simulink model "Passive_Balance"  (R2020a)
settings: Solver=FixedStepDiscrete  StartTime=0.0  StopTime=1  FixedStep=1e-3  RelTol=1e-3
libraries: simulink x1
settings Model: Creator=Administrator  LastModifiedBy=Administrator
settings OptimizationCC: DefaultParameterBehavior=Inlined  EnhancedBackFolding=on  PassReuseOutputArgsAs=Individual arguments  ZeroExternalMemoryAtStartup=off  ZeroInternalMemoryAtStartup=off  OptimizeBlockOrder=speed  DifferentSizesBufferReuse=on  OptimizationCustomize=off  EfficientTunableParamExpr=on
settings DebuggingCC: ParameterTunabilityLossMsg=error
settings HardwareCC: ProdBitPerPointer=32  ProdBitPerSizeT=32  ProdBitPerPtrDiffT=32  ProdLargestAtomicInteger=Long  ProdLargestAtomicFloat=Double  ProdWordSize=32  ProdHWDeviceType=ARM Compatible->ARM Cortex
settings SFSimCC: MATLABDynamicMemAlloc=off
settings RTWCC: SystemTargetFile=ert.tlc  TemplateMakefile=ert_default_tmf
settings CodeAppCC: ForceParamTrailComments=on  IgnoreCustomStorageClasses=off  OperatorAnnotations=on  SimulinkDataObjDesc=on  SFDataObjDesc=on  InsertBlockDesc=on
settings ERTTargetCC: TargetLangStandard=C99 (ISO)  GenerateSampleERTMain=on  InlinedParameterPlacement=NonHierarchical  ERTCustomFileTemplate=example_file_process.tlc

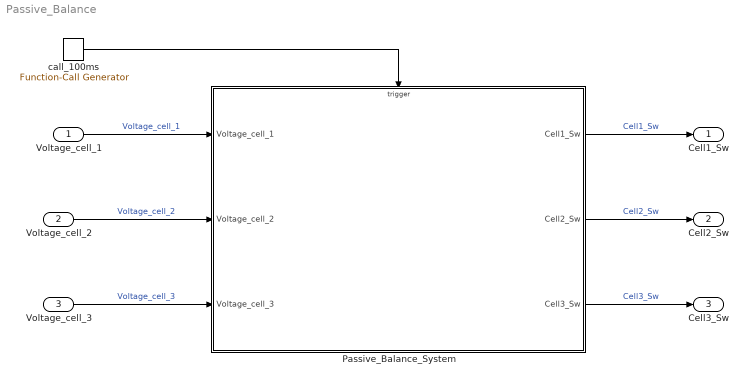
== system Passive_Balance ==
  Voltage_cell_1 : Inport
  Voltage_cell_2 : Inport  Port=2
  Voltage_cell_3 : Inport  Port=3
  Passive_Balance_System : Subsystem
  call_100ms : simulink/Ports & Subsystems/Function-Call Generator  sample_time=1e-3  numberOfIterations=1
  Cell1_Sw : Outport
  Cell2_Sw : Outport  Port=2
  Cell3_Sw : Outport  Port=3
  wires:
  call_100ms/1 -> Passive_Balance_System/Trigger
  Voltage_cell_3/1 -> Passive_Balance_System/3(Voltage_cell_3)  "Voltage_cell_3"
  Voltage_cell_2/1 -> Passive_Balance_System/2(Voltage_cell_2)  "Voltage_cell_2"
  Passive_Balance_System/3(Cell3_Sw) -> Cell3_Sw/1  "Cell3_Sw"
  Passive_Balance_System/2(Cell2_Sw) -> Cell2_Sw/1  "Cell2_Sw"
  Passive_Balance_System/1(Cell1_Sw) -> Cell1_Sw/1  "Cell1_Sw"
  Voltage_cell_1/1 -> Passive_Balance_System/1(Voltage_cell_1)  "Voltage_cell_1"

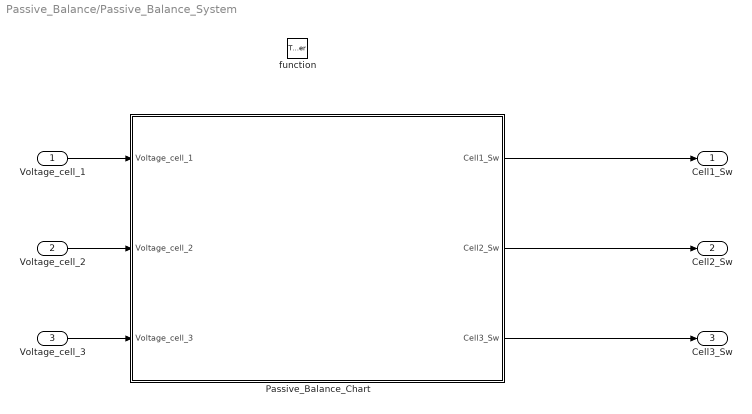
== system Passive_Balance/Passive_Balance_System ==
  Voltage_cell_1 : Inport
  Voltage_cell_2 : Inport  Port=2
  Voltage_cell_3 : Inport  Port=3
  function : TriggerPort  TriggerType=function-call  VariantControl=Variant  StatesWhenEnabling=reset
  Passive_Balance_Chart : Stateflow chart  TreatAsAtomicUnit=on
  Cell1_Sw : Outport
  Cell2_Sw : Outport  Port=2
  Cell3_Sw : Outport  Port=3
  wires:
  Voltage_cell_2/1 -> Passive_Balance_Chart/2(Voltage_cell_2)
  Voltage_cell_1/1 -> Passive_Balance_Chart/1(Voltage_cell_1)
  Voltage_cell_3/1 -> Passive_Balance_Chart/3(Voltage_cell_3)
  Passive_Balance_Chart/1(Cell1_Sw) -> Cell1_Sw/1
  Passive_Balance_Chart/3(Cell3_Sw) -> Cell3_Sw/1
  Passive_Balance_Chart/2(Cell2_Sw) -> Cell2_Sw/1

== stateflow chart Passive_Balance/Passive_Balance_System/Passive_Balance_Chart ==
  state Balancer
    state Mange_Sw
      state Mode_A
        entry:
        Cell2_Sw=1;
        Cell3_Sw=1;
        during:
        Need_No_Balance();
        equality();
        ex:
        Cell2_Sw=1;
        Cell3_Sw=1;
      state Mode_C
        entry:
        Cell1_Sw=1;
        Cell3_Sw=1;
        during:
        Need_No_Balance();
        equality();
        ex:
        Cell1_Sw=1;
        Cell3_Sw=1;
      state Mode_B
        entry:
        Cell2_Sw=1;
        Cell1_Sw=1;
        during:
        Need_No_Balance();
        equality();
        ex:
        Cell2_Sw=0;
        Cell1_Sw=0;
      (junction 175) -> (junction 147)
      (junction 147) -> (junction 151) [order 1] : [Lowest_B==1]
      (junction 147) -> (junction 153) [order 2] : [Lowest_B==3]
      (junction 151) -> Mode_A
      (junction 147) -> Mode_C [order 3] : [Lowest_B==2]
      (junction 153) -> Mode_B
    state All_Balanced
      entry:
      Need_No_Balance();
      during:
      Need_No_Balance();
      State_Cell1();
      State_Cell2();
      State_Cell3();
    (default) -> All_Balanced
    All_Balanced -> (junction 175) : [state==0 ]
    Mange_Sw -> All_Balanced : [state==1 ]
  state equality [function]
    (default) -> (junction 447)
    (junction 447) -> (junction 450) [order 3] : [Lowest_B==2]
    (junction 447) -> (junction 449) [order 2] : [Lowest_B==3]
    (junction 447) -> (junction 483) [order 1] : [Lowest_B==1]
    (junction 449) -> (junction 465)
    (junction 450) -> (junction 521)
    (junction 465) -> (junction 466) [order 1] : [Voltage_cell_1==Voltage_cell_3]
    (junction 465) -> (junction 467) [order 2]
    (junction 466) -> (junction 471) : {Cell1_Sw=0;}
    (junction 521) -> (junction 519) [order 1] : [Voltage_cell_1==Voltage_cell_2]
    (junction 483) -> (junction 477) [order 1] : [Voltage_cell_1==Voltage_cell_3]
    (junction 521) -> (junction 517) [order 2]
    (junction 483) -> (junction 480) [order 2]
    (junction 519) -> (junction 526) : {Cell1_Sw=0;}
    (junction 477) -> (junction 491) : {Cell3_Sw=0;}
    (junction 467) -> (junction 468) [order 1] : [Voltage_cell_2==Voltage_cell_3]
    (junction 467) -> (junction 469) [order 2]
    (junction 468) -> (junction 470) : {Cell2_Sw=0;}
    (junction 517) -> (junction 529) [order 1] : [Voltage_cell_2==Voltage_cell_3]
    (junction 480) -> (junction 487) [order 1] : [Voltage_cell_2==Voltage_cell_1]
    (junction 517) -> (junction 528) [order 2]
    (junction 529) -> (junction 520) : {Cell3_Sw=0;}
    (junction 480) -> (junction 489) [order 2]
    (junction 487) -> (junction 482) : {Cell2_Sw=0;}
    (junction 470) -> (junction 469)
    (junction 471) -> (junction 470)
    (junction 469) -> (junction 472)
    (junction 520) -> (junction 528)
    (junction 526) -> (junction 520)
    (junction 482) -> (junction 489)
    (junction 491) -> (junction 482)
    (junction 528) -> (junction 515)
    (junction 489) -> (junction 478)
  state Need_No_Balance [function]
    (default) -> (junction 195)
    (junction 195) -> (junction 196) [order 1] : [Voltage_cell_1==Voltage_cell_2 && Voltage_cell_1==Voltage_cell_3]
    (junction 195) -> (junction 197) [order 2] : {state=0;}
    (junction 196) -> (junction 198) : {state=1;}
    (junction 198) -> (junction 197)
    (junction 197) -> (junction 199)
  state State_Cell1 [function]
    (default) -> (junction 58) : [Voltage_cell_1>=Voltage_cell_2>=Voltage_cell_3]
    (junction 58) -> (junction 59) [order 1] : [Voltage_cell_2>=Voltage_cell_3]
    (junction 58) -> (junction 60) [order 2]
    (junction 59) -> (junction 64) : {Lowest_B=3;}
    (junction 60) -> (junction 61) [order 1] : [Voltage_cell_3>=Voltage_cell_2]
    (junction 60) -> (junction 62) [order 2]
    (junction 61) -> (junction 63) : {Lowest_B=2;}
    (junction 63) -> (junction 62)
    (junction 64) -> (junction 63)
    (junction 62) -> (junction 65)
  state State_Cell2 [function]
    (default) -> (junction 69) : [Voltage_cell_2>=Voltage_cell_1>=Voltage_cell_3]
    (junction 69) -> (junction 70) [order 1] : [Voltage_cell_1>=Voltage_cell_3]
    (junction 69) -> (junction 68) [order 2]
    (junction 70) -> (junction 73) : {Lowest_B=3;}
    (junction 68) -> (junction 72) [order 1] : [Voltage_cell_3>=Voltage_cell_1]
    (junction 68) -> (junction 66) [order 2]
    (junction 72) -> (junction 75) : {Lowest_B=1;}
    (junction 75) -> (junction 66)
    (junction 73) -> (junction 75)
    (junction 66) -> (junction 76)
  state State_Cell3 [function]
    (default) -> (junction 90) : [Voltage_cell_3>=Voltage_cell_1>=Voltage_cell_2]
    (junction 90) -> (junction 86) [order 1] : [Voltage_cell_1>=Voltage_cell_2]
    (junction 90) -> (junction 91) [order 2]
    (junction 86) -> (junction 94) : {Lowest_B=2;}
    (junction 91) -> (junction 87) [order 1] : [Voltage_cell_2>=Voltage_cell_1]
    (junction 91) -> (junction 89) [order 2]
    (junction 87) -> (junction 92) : {Lowest_B=1;}
    (junction 92) -> (junction 89)
    (junction 94) -> (junction 92)
    (junction 89) -> (junction 96)
  (default) -> Balancer
  data: Voltage_cell_1 input; Voltage_cell_2 input; Voltage_cell_3 input; Lowest_B local double; state local double =0; Cell1_Sw output boolean; Cell2_Sw output boolean; Cell3_Sw output boolean
